simulink model "SGN_guidance_simulator"  (R2025b)
settings: Solver=ode45  StartTime=0.0  StopTime=50  MaxStep=0.01  RelTol=1e-3  EnableMultiTasking=on
values from neighbouring files (symbols this model uses):
  BETA_INI = 225*pi/180    (= 3.92699081699)    [SGN_drone_challenge_ini.m]
  GUIDANCE_MODE = 2    [SGN_drone_challenge_ini.m]
  GUIDE_SEL = 0    [SGN_drone_challenge_ini.m]
  LOS_INI = atan2(YT_INI - YM_INI, XT_INI - XM_INI)    [SGN_drone_challenge_ini.m]
  MAX_ACC = 0.25    [SGN_drone_challenge_ini.m]
  RTOL = 0.01    [SGN_drone_challenge_ini.m]
  SGN_GUIDANCE_PARAMS = [ ... (first row only)    [SGN_drone_challenge_ini.m]
  Tautopilot = 0.35    [SGN_drone_challenge_ini.m]
  VT = 0.2    [SGN_drone_challenge_ini.m]
  VXM_INI = VM*cos(GAMMA_INI)    [SGN_drone_challenge_ini.m]
  VYM_INI = VM*sin(GAMMA_INI)    [SGN_drone_challenge_ini.m]
  XM_INI = -1.0    (= -1)    [SGN_drone_challenge_ini.m]
  XT_INI = 1.0    (= 1)    [SGN_drone_challenge_ini.m]
  YM_INI = -1.0    (= -1)    [SGN_drone_challenge_ini.m]
  YT_INI = 0.0    (= 0)    [SGN_drone_challenge_ini.m]
settings Model: Creator=Lorenzo  LastModifiedBy=roly2
settings SolverCC: ZeroCrossAlgorithm=Non-adaptive  AlgebraicLoopSolver=TrustRegion
settings DataIOCC: LimitDataPoints=on  SaveFormat=Array  SignalLoggingSaveFormat=ModelDataLogs  ReturnWorkspaceOutputs=off
settings OptimizationCC: ExpressionDepthLimit=2147483647.0  InitFltsAndDblsToZero=on  LifeSpan=inf
settings DebuggingCC: SaveWithParameterizedLinksMsg=none  UnderspecifiedInitializationDetection=Classic  MergeDetectMultiDrivingBlocksExec=none  SolverPrmCheckMsg=warning  FcnCallInpInsideContextMsg=warning  UnconnectedInputMsg=warning  UnconnectedOutputMsg=warning  UnconnectedLineMsg=warning  StateNameClashWarn=warning  SFUnexpectedBacktrackingDiag=warning  SFNoUnconditionalDefaultTransitionDiag=warning  SFExecutionAtInitializationDiag=none  ArithmeticOperatorsInVariantConditions=warning
settings HardwareCC: ProdBitPerPointer=32.0  ProdBitPerSizeT=32.0  ProdBitPerPtrDiffT=32.0  ProdLargestAtomicFloat=None  ProdIntDivRoundTo=Undefined  ProdEndianess=Unspecified  ProdWordSize=32.0  ProdHWDeviceType=32-bit Generic
settings ModelReferenceCC: PropagateSignalLabelsOutOfModel=off
settings RTWCC: GPUComputeCapability=3.5
settings CodeAppCC: StateflowObjectComments=on
settings GRTTargetCC: TargetFcnLib=ansi_tfl_tmw.mat  TargetLangStandard=C89/C90 (ANSI)  CombineOutputUpdateFcns=off  GRTInterface=on
settings ConfigComp: CovMetricSettings=dw  CovSaveCumulativeToWorkspaceVar=on  CovSaveSingleToWorkspaceVar=on

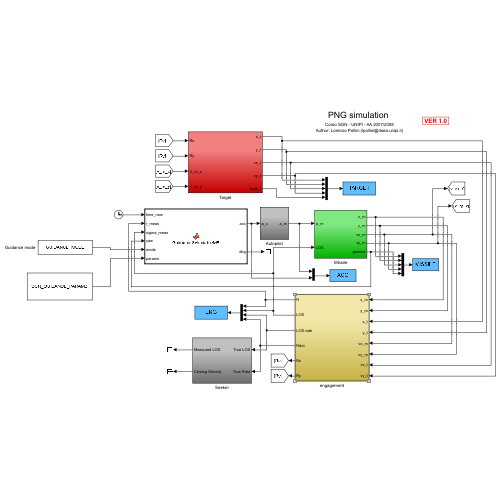
[thumbnail: Simulink's stored preview of the top-level diagram]
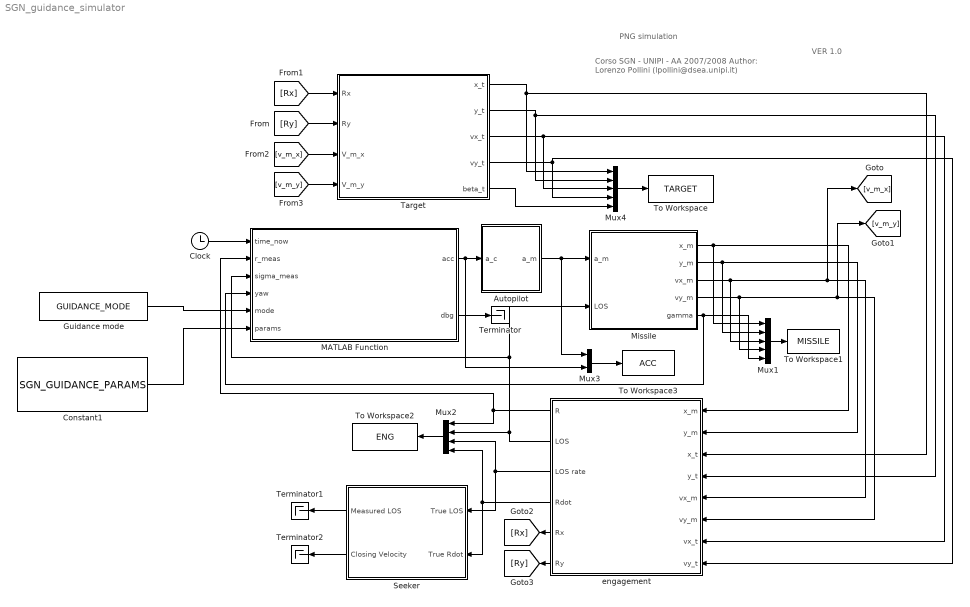
== system SGN_guidance_simulator ==
  note: PNG simulation
  note: Corso SGN - UNIPI - AA 2007/2008
      | Author: Lorenzo Pollini (lpollini@dsea.unipi.it)
  note: VER 1.0
  Autopilot : Subsystem
  Clock : Clock
  Constant1 : Constant  Value=SGN_GUIDANCE_PARAMS
  Guidance mode : Constant  Value=GUIDANCE_MODE
  MATLAB Function : MATLAB Function  TreatAsAtomicUnit=on
  Missile : Subsystem
  Mux1 : Mux  Inputs=5
  Mux2 : Mux
  Mux3 : Mux  Inputs=2
  Mux4 : Mux  Inputs=5
  Seeker : Subsystem
  Target : Subsystem
  Terminator : Terminator
  Terminator1 : Terminator
  Terminator2 : Terminator
  To Workspace : ToWorkspace  VariableName=TARGET  SaveFormat=Structure With Time  SampleTime=-1
  To Workspace1 : ToWorkspace  VariableName=MISSILE  SaveFormat=Structure With Time  SampleTime=-1
  To Workspace2 : ToWorkspace  VariableName=ENG  SaveFormat=Structure With Time  SampleTime=-1
  To Workspace3 : ToWorkspace  VariableName=ACC  SaveFormat=Structure With Time  SampleTime=-1
  engagement : Subsystem
  wires:
  Target/1(x_t) -> engagement/3(x_t), Mux4/1
  Target/2(y_t) -> engagement/4(y_t), Mux4/2
  Target/3(vx_t) -> engagement/7(vx_t), Mux4/3
  Target/4(vy_t) -> engagement/8(vy_t), Mux4/4
  Missile/1(x_m) -> engagement/1(x_m), Mux1/1
  Missile/2(y_m) -> engagement/2(y_m), Mux1/2
  Missile/3(vx_m) -> [v_m_x], engagement/5(vx_m), Mux1/3
  Missile/4(vy_m) -> Mux1/4, [v_m_y], engagement/6(vy_m)
  engagement/2(LOS) -> MATLAB Function/3(sigma_meas), Missile/2(LOS), Mux2/2
  engagement/3(LOS rate) -> Seeker/1(True LOS), Mux2/3
  engagement/4(Rdot) -> Seeker/2(True Rdot), Mux2/4
  MATLAB Function/1(acc) -> Mux3/2, Autopilot/1(a_c)
  Mux4/1 -> To Workspace/1
  Mux1/1 -> To Workspace1/1
  Mux2/1 -> To Workspace2/1
  engagement/1(R) -> Mux2/1, MATLAB Function/2(r_meas)
  Autopilot/1(a_m) -> Missile/1(a_m), Mux3/1
  Missile/5(gamma) -> MATLAB Function/4(yaw), Mux1/5
  Mux3/1 -> To Workspace3/1
  Target/5(beta_t) -> Mux4/5
  Clock/1 -> MATLAB Function/1(time_now)
  MATLAB Function/2(dbg) -> Terminator/1
  Guidance mode/1 -> MATLAB Function/5(mode)
  Constant1/1 -> MATLAB Function/6(params)
  Seeker/1(Measured LOS) -> Terminator1/1
  Seeker/2(Closing Velocity) -> Terminator2/1
  [Rx] -> Target/1(Rx)
  [Ry] -> Target/2(Ry)
  [v_m_x] -> Target/3(V_m_x)
  [v_m_y] -> Target/4(V_m_y)
  engagement/5(Rx) -> [Rx]
  engagement/6(Ry) -> [Ry]

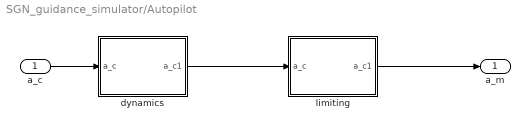
== system SGN_guidance_simulator/Autopilot ==
  a_c : Inport
  dynamics : Subsystem
  limiting : Subsystem
  a_m : Outport
  wires:
  a_c/1 -> dynamics/1(a_c)
  dynamics/1(a_c1) -> limiting/1(a_c)
  limiting/1(a_c1) -> a_m/1

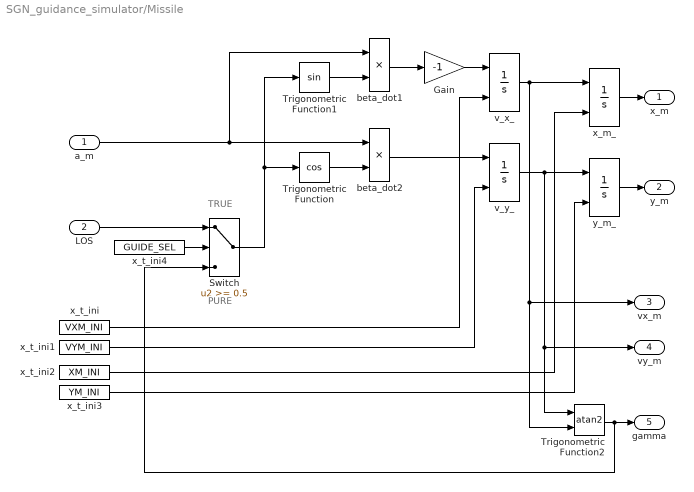
== system SGN_guidance_simulator/Missile ==
  note: TRUE
  note: PURE
  a_m : Inport
  LOS : Inport  Port=2
  Gain : Gain  Gain=-1
  Switch : Switch  Threshold=0.5  SaturateOnIntegerOverflow=off  InputSameDT=off
  Trigonometric Function : Trigonometry  Operator=cos
  Trigonometric Function1 : Trigonometry
  Trigonometric Function2 : Trigonometry  Operator=atan2
  beta_dot1 : Product  Inputs=**
  beta_dot2 : Product  Inputs=**
  v_x_ : Integrator  InitialConditionSource=external
  v_y_ : Integrator  InitialConditionSource=external
  x_m_ : Integrator  InitialConditionSource=external
  x_t_ini : Constant  Value=VXM_INI
  x_t_ini1 : Constant  Value=VYM_INI
  x_t_ini2 : Constant  Value=XM_INI
  x_t_ini3 : Constant  Value=YM_INI
  x_t_ini4 : Constant  Value=GUIDE_SEL
  y_m_ : Integrator  InitialConditionSource=external
  x_m : Outport
  y_m : Outport  Port=2
  vx_m : Outport  Port=3
  vy_m : Outport  Port=4
  gamma : Outport  Port=5
  wires:
  Trigonometric Function/1 -> beta_dot2/2
  beta_dot1/1 -> Gain/1
  Trigonometric Function1/1 -> beta_dot1/2
  y_m_/1 -> y_m/1
  x_m_/1 -> x_m/1
  v_x_/1 -> x_m_/1, vx_m/1, Trigonometric Function2/2
  v_y_/1 -> y_m_/1, vy_m/1, Trigonometric Function2/1
  Gain/1 -> v_x_/1
  a_m/1 -> beta_dot1/1, beta_dot2/1
  beta_dot2/1 -> v_y_/1
  x_t_ini/1 -> v_x_/2
  x_t_ini1/1 -> v_y_/2
  x_t_ini2/1 -> x_m_/2
  x_t_ini3/1 -> y_m_/2
  Trigonometric Function2/1 -> gamma/1, Switch/3
  LOS/1 -> Switch/1
  Switch/1 -> Trigonometric Function1/1, Trigonometric Function/1
  x_t_ini4/1 -> Switch/2

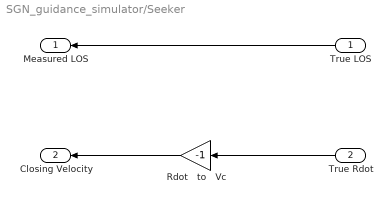
== system SGN_guidance_simulator/Seeker ==
  True LOS : Inport
  True Rdot : Inport  Port=2
  Rdot   to   Vc : Gain  Gain=-1
  Measured LOS : Outport
  Closing Velocity : Outport  Port=2
  wires:
  True LOS/1 -> Measured LOS/1
  Rdot   to   Vc/1 -> Closing Velocity/1
  True Rdot/1 -> Rdot   to   Vc/1

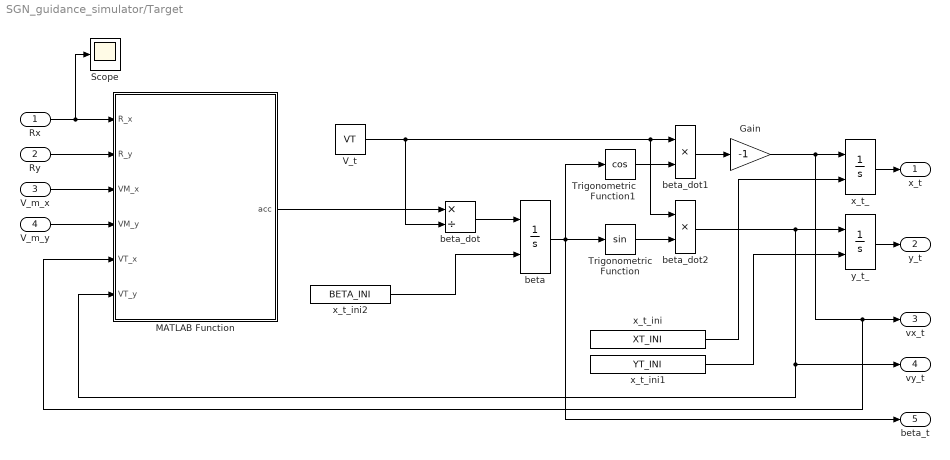
== system SGN_guidance_simulator/Target ==
  Rx : Inport
  Ry : Inport  Port=2
  V_m_x : Inport  Port=3
  V_m_y : Inport  Port=4
  Gain : Gain  Gain=-1
  MATLAB Function : MATLAB Function  TreatAsAtomicUnit=on
  Scope : Scope
      settings: ActiveDisplayYMinimum=-1  ActiveDisplayYMaximum=1
  Trigonometric Function : Trigonometry
  Trigonometric Function1 : Trigonometry  Operator=cos
  V_t : Constant  Value=VT
  beta : Integrator  InitialConditionSource=external
  beta_dot : Product  Inputs=*/
  beta_dot1 : Product  Inputs=**
  beta_dot2 : Product  Inputs=**
  x_t_ : Integrator  InitialConditionSource=external
  x_t_ini : Constant  Value=XT_INI
  x_t_ini1 : Constant  Value=YT_INI
  x_t_ini2 : Constant  Value=BETA_INI
  y_t_ : Integrator  InitialConditionSource=external
  x_t : Outport
  y_t : Outport  Port=2
  vx_t : Outport  Port=3
  vy_t : Outport  Port=4
  beta_t : Outport  Port=5
  wires:
  V_t/1 -> beta_dot1/1, beta_dot2/1, beta_dot/2
  beta_dot/1 -> beta/1
  beta/1 -> Trigonometric Function/1, Trigonometric Function1/1, beta_t/1
  x_t_ini2/1 -> beta/2
  x_t_/1 -> x_t/1
  y_t_/1 -> y_t/1
  Trigonometric Function1/1 -> beta_dot1/2
  beta_dot1/1 -> Gain/1
  Trigonometric Function/1 -> beta_dot2/2
  beta_dot2/1 -> y_t_/1, MATLAB Function/6(VT_y), vy_t/1
  Gain/1 -> x_t_/1, MATLAB Function/5(VT_x), vx_t/1
  x_t_ini1/1 -> y_t_/2
  x_t_ini/1 -> x_t_/2
  MATLAB Function/1(acc) -> beta_dot/1
  Rx/1 -> Scope/1, MATLAB Function/1(R_x)
  Ry/1 -> MATLAB Function/2(R_y)
  V_m_x/1 -> MATLAB Function/3(VM_x)
  V_m_y/1 -> MATLAB Function/4(VM_y)

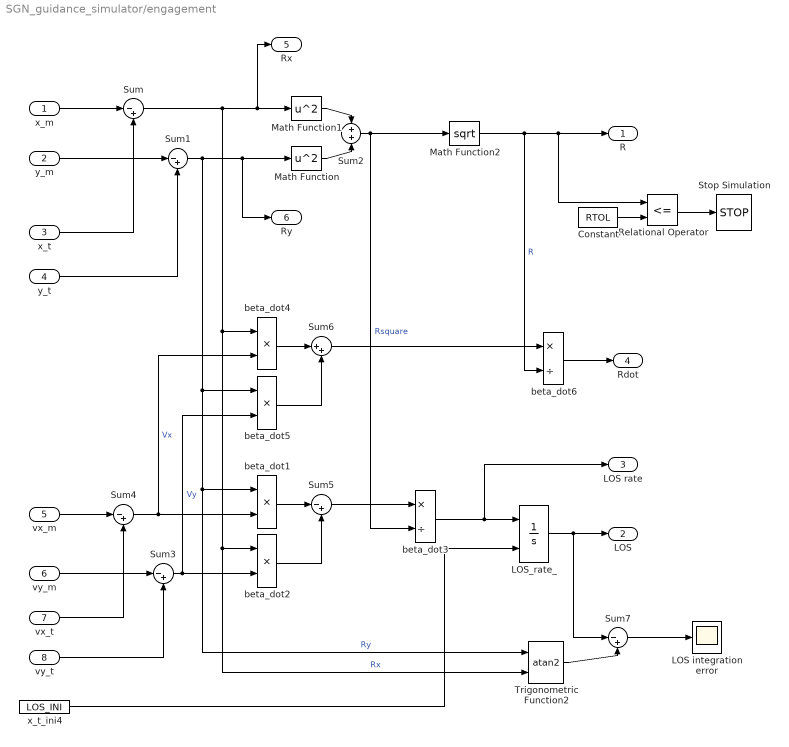
== system SGN_guidance_simulator/engagement ==
  x_m : Inport
  y_m : Inport  Port=2
  x_t : Inport  Port=3
  y_t : Inport  Port=4
  vx_m : Inport  Port=5
  vy_m : Inport  Port=6
  vx_t : Inport  Port=7
  vy_t : Inport  Port=8
  Constant : Constant  Value=RTOL
  LOS integration error : Scope
  LOS_rate_ : Integrator  InitialConditionSource=external
  Math Function : Math  Operator=square  SignedPower=on
  Math Function1 : Math  Operator=square  SignedPower=on
  Math Function2 : Math  Operator=sqrt  SignedPower=on
  Relational Operator : RelationalOperator  Operator=<=  OutDataTypeStr=boolean  InputSameDT=off
  Stop Simulation : Stop
  Sum{,1,3..5,7} (6 alike) : Sum  Inputs=|-+
  Sum2 : Sum  Inputs=+|+
  Sum6 : Sum  Inputs=|++
  Trigonometric Function2 : Trigonometry  Operator=atan2
  beta_dot{1..2,4..5} (4 alike) : Product  Inputs=**
  beta_dot3 : Product  Inputs=*/
  beta_dot6 : Product  Inputs=*/
  x_t_ini4 : Constant  Value=LOS_INI
  R : Outport
  LOS : Outport  Port=2
  LOS rate : Outport  Port=3
  Rdot : Outport  Port=4
  Rx : Outport  Port=5
  Ry : Outport  Port=6
  wires:
  x_t_ini4/1 -> LOS_rate_/2
  x_m/1 -> Sum/1
  x_t/1 -> Sum/2
  y_m/1 -> Sum1/1
  y_t/1 -> Sum1/2
  Sum/1 -> Rx/1, Math Function1/1, beta_dot4/1, beta_dot2/1, Trigonometric Function2/2  "Rx"
  Sum1/1 -> Ry/1, Math Function/1, beta_dot5/1, beta_dot1/1, Trigonometric Function2/1  "Ry"
  Math Function1/1 -> Sum2/1
  Math Function/1 -> Sum2/2
  Sum2/1 -> Math Function2/1, beta_dot3/2  "Rsquare"
  Math Function2/1 -> beta_dot6/2, R/1, Relational Operator/1  "R"
  vx_m/1 -> Sum4/1
  vx_t/1 -> Sum4/2
  vy_m/1 -> Sum3/1
  vy_t/1 -> Sum3/2
  Sum4/1 -> beta_dot1/2, beta_dot4/2  "Vx"
  Sum3/1 -> beta_dot2/2, beta_dot5/2  "Vy"
  beta_dot1/1 -> Sum5/1
  beta_dot2/1 -> Sum5/2
  Sum5/1 -> beta_dot3/1
  beta_dot3/1 -> LOS_rate_/1, LOS rate/1
  LOS_rate_/1 -> LOS/1, Sum7/1
  beta_dot4/1 -> Sum6/1
  beta_dot5/1 -> Sum6/2
  Sum6/1 -> beta_dot6/1
  beta_dot6/1 -> Rdot/1
  Constant/1 -> Relational Operator/2
  Relational Operator/1 -> Stop Simulation/1
  Trigonometric Function2/1 -> Sum7/2
  Sum7/1 -> LOS integration error/1

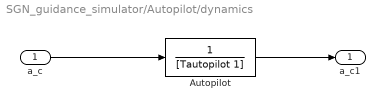
== system SGN_guidance_simulator/Autopilot/dynamics ==
  a_c : Inport
  Autopilot : TransferFcn  Denominator=[Tautopilot 1]
  a_c1 : Outport
  wires:
  a_c/1 -> Autopilot/1
  Autopilot/1 -> a_c1/1

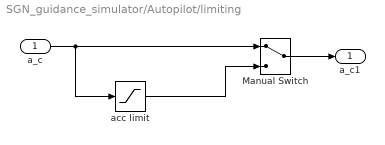
== system SGN_guidance_simulator/Autopilot/limiting ==
  a_c : Inport
  Manual Switch : ManualSwitch
  acc limit : Saturate  UpperLimit=MAX_ACC  LowerLimit=-MAX_ACC
  a_c1 : Outport
  wires:
  Manual Switch/1 -> a_c1/1
  a_c/1 -> Manual Switch/1, acc limit/1
  acc limit/1 -> Manual Switch/2

== matlab function SGN_guidance_simulator/Target/MATLAB Function ==
  data: R_x input; acc output; R_y input; VM_x input; VM_y input; VT_x input; VT_y input
function acc = evadi_missile_simulink(R_x, R_y, VM_x, VM_y, VT_x, VT_y)
%#codegen
%
% R_x, R_y   : posizione relativa target - missile
% VM_x, VM_y : velocità missile
% VT_x, VT_y : velocità target
%
% acc = +0.2  -> virata a sinistra
% acc = -0.2  -> virata a destra
% acc =  0.0  -> nessuna manovra evasiva
 
    % Parametri
    soglia_distanza = 0.2;   % [m]
    acc_evasiva     = 0.2;   % [m/s^2]
 
    eps_r     = 1e-9;
    eps_cross = 1e-9;
    eps_vc    = 1e-6;
 
    % Default
    acc = 0.0;
 
    % Distanza missile-target
    distanza = sqrt(R_x^2 + R_y^2);
 
    % Evita problemi numerici se missile e target sono quasi sovrapposti
    if distanza < eps_r
        return;
    end
 
    % Velocità relativa coerente con R = P_T - P_M
    V_rel_x = VT_x - VM_x;
    V_rel_y = VT_y - VM_y;
 
    % Derivata della distanza
    R_dot = (R_x * V_rel_x + R_y * V_rel_y) / distanza;
 
    % Closing velocity: positiva se il missile si sta avvicinando
    Vc = -R_dot;
 
    % Se il missile è lontano oppure non si sta avvicinando, non evado
    if distanza > soglia_distanza || Vc <= eps_vc
        acc = 0.0;
        return;
    end
 
    % Prodotto vettoriale 2D tra R e V_rel
    % Serve a capire da che lato sta "tagliando" il missile
    cross_z = R_x * V_rel_y - R_y * V_rel_x;
 
    % Scelta del verso di virata
    %
    % Manteniamo la stessa logica del tuo codice originale:
    % cross_z >= 0 -> normale destra  [ R_y, -R_x] -> acc negativa
    % cross_z <  0 -> normale sinistra[-R_y,  R_x] -> acc positiva
 
    if cross_z > eps_cross
        acc = -acc_evasiva;      % vira a destra
    elseif cross_z < -eps_cross
        acc = +acc_evasiva;      % vira a sinistra
    else
        % Caso quasi frontale o quasi perfettamente allineato:
        % il lato è ambiguo, scelgo una manovra deterministica
        acc = +acc_evasiva;
    end
end
% function acc_t = target_int(R, Ry)
% 
% if (R < 0.3)
%     if (sign(Ry) > 0)
%         acc_t = -0.2;
%     else 
%         acc_t = 0.2;
%     end
% else
%     acc_t = 0.0;
% end

== matlab function SGN_guidance_simulator/MATLAB Function ==
  settings: updateMethod=DISCRETE
  data: time_now input; acc output; r_meas input; sigma_meas input; yaw input; dbg output; mode input; params input
function [acc, dbg] = GuidanceSelectableMF(time_now, r_meas, sigma_meas, yaw, mode, params)
% MATLAB Function block code.
%
% mode:
%   1 pursuit
%   2 PNG
%   3 APNG
%   4 adaptive
%
% params: 16x1 vector
%
% This block is code-generation-safe: no try, no evalin.

%#codegen

reset = false;

[acc, dbg] = sgn_guidance_core(mode, time_now, r_meas, sigma_meas, yaw, reset, params);

end
